simulink model "robot_ver_wheel"  (R2022b)
settings: Solver=VariableStepAuto  StartTime=0.0  StopTime=10  RelTol=1e-3
values from neighbouring files (symbols this model uses):
  m = 3.0    (= 3)    [robot_obstacle_parameters.m]
settings Model: Creator=rplatz  LastModifiedBy=rplatz
settings ModelReferenceCC: EnableRefExpFcnMdlSchedulingChecks=on

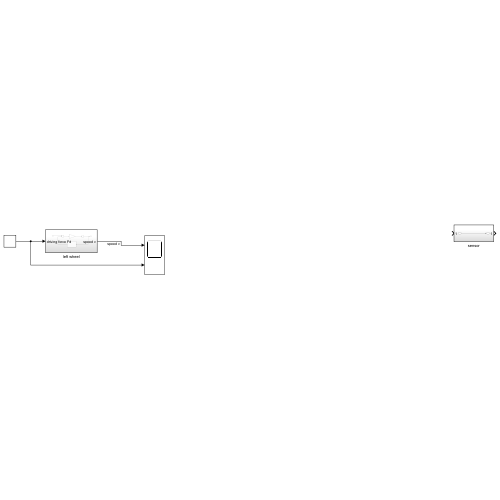
[thumbnail: Simulink's stored preview of the top-level diagram]
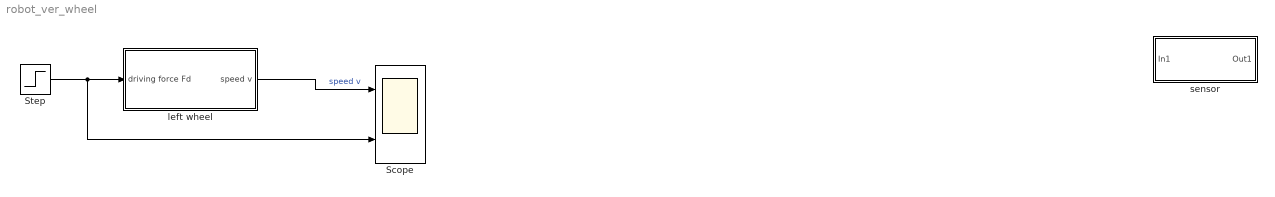
== system robot_ver_wheel ==
  Scope : Scope  NumInputPorts=2
  Step : Step  SampleTime=0
  left wheel : Subsystem
  sensor : Subsystem
  wires:
  Step/1 -> Scope/2, left wheel/1(driving force Fd)
  left wheel/1(speed v) -> Scope/1  "speed v"

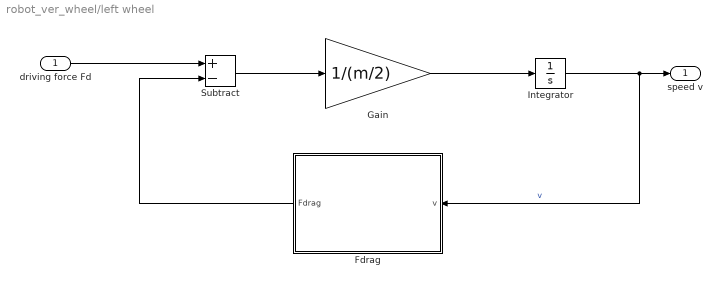
== system robot_ver_wheel/left wheel ==
  driving force Fd : Inport
  Fdrag : MATLAB Function  TreatAsAtomicUnit=on
  Gain : Gain  Gain=1/(m/2)
  Integrator : Integrator
  Subtract : Sum  Inputs=+-
  speed v : Outport
  wires:
  driving force Fd/1 -> Subtract/1
  Fdrag/1(Fdrag) -> Subtract/2
  Subtract/1 -> Gain/1
  Gain/1 -> Integrator/1
  Integrator/1 -> Fdrag/1(v), speed v/1  "v"

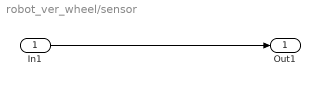
== system robot_ver_wheel/sensor ==
  In1 : Inport
  Out1 : Outport
  wires:
  In1/1 -> Out1/1

== matlab function robot_ver_wheel/left wheel/Fdrag ==
  data: v input; Fdrag output; k_drag parameter
function Fdrag = get_Fdrag(v,k_drag)

Fdrag = k_drag*v*abs(v);
